simulink model "simpleTreeDiff"  (R2024b)
settings: Solver=VariableStepAuto  StartTime=0.0  StopTime=10.0  RelTol=1e-3
settings Model: Creator=neham  LastModifiedBy=neham

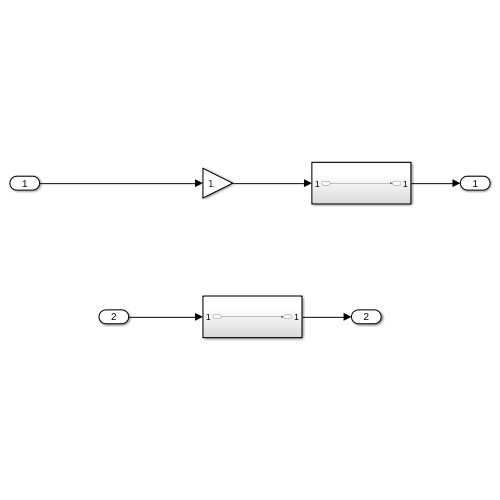
[thumbnail: Simulink's stored preview of the top-level diagram]
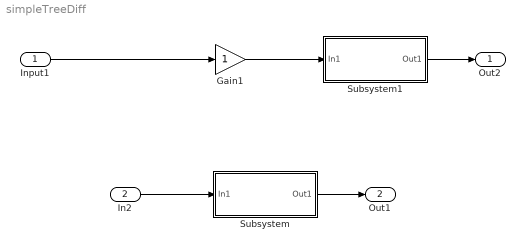
== system simpleTreeDiff ==
  Input1 : Inport
  In2 : Inport  Port=2
  Gain1 : Gain
  Subsystem : Subsystem
  Subsystem1 : Subsystem
  Out2 : Outport
  Out1 : Outport  Port=2
  wires:
  Input1/1 -> Gain1/1
  Gain1/1 -> Subsystem1/1(In1)
  In2/1 -> Subsystem/1(In1)
  Subsystem1/1(Out1) -> Out2/1
  Subsystem/1(Out1) -> Out1/1

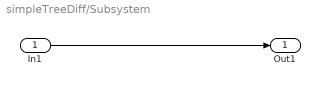
== system simpleTreeDiff/Subsystem ==
  In1 : Inport
  Out1 : Outport
  wires:
  In1/1 -> Out1/1

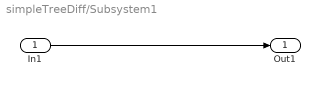
== system simpleTreeDiff/Subsystem1 ==
  In1 : Inport
  Out1 : Outport
  wires:
  In1/1 -> Out1/1
